simulink subsystem "Plot_Performance"  (R2024b)
settings: Solver=VariableStepAuto  StartTime=0.0  StopTime=10.0  RelTol=1e-3
values from neighbouring files (symbols this model uses):
  BBOD5 = 2    [Run_algo.m]    (also in Run_interpolation.m; perf_plant.m; perf_plant_v3.m; run_bsm1_PIANN.m)
  BNKj_new = 30    [Run_algo.m]    (also in Run_interpolation.m; perf_plant.m; perf_plant_v3.m; run_bsm1_PIANN.m)
  BNO_new = 10    [Run_algo.m]    (also in Run_interpolation.m; perf_plant.m; perf_plant_v3.m; run_bsm1_PIANN.m)
  BSS = 2    [Run_algo.m]    (also in Run_interpolation.m; perf_plant.m; perf_plant_v3.m; run_bsm1_PIANN.m)
  SampleTime = 0.0001    [Run_algo.m]    (also in Run_interpolation.m)
undefined symbols (not defined in the file or in its folder): f_P, i_XB, i_XP
settings Model: Creator=1630327  LastModifiedBy=1630327

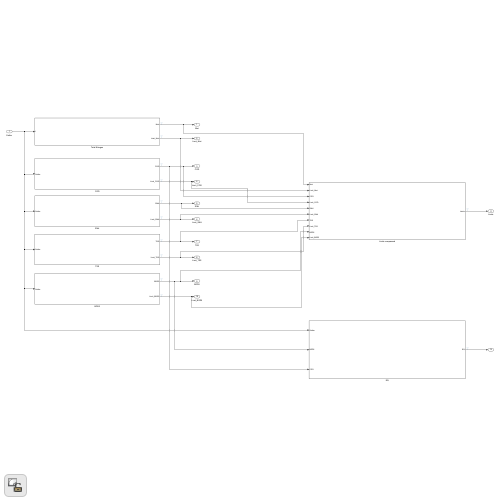
[thumbnail: Simulink's stored preview of the top-level diagram]
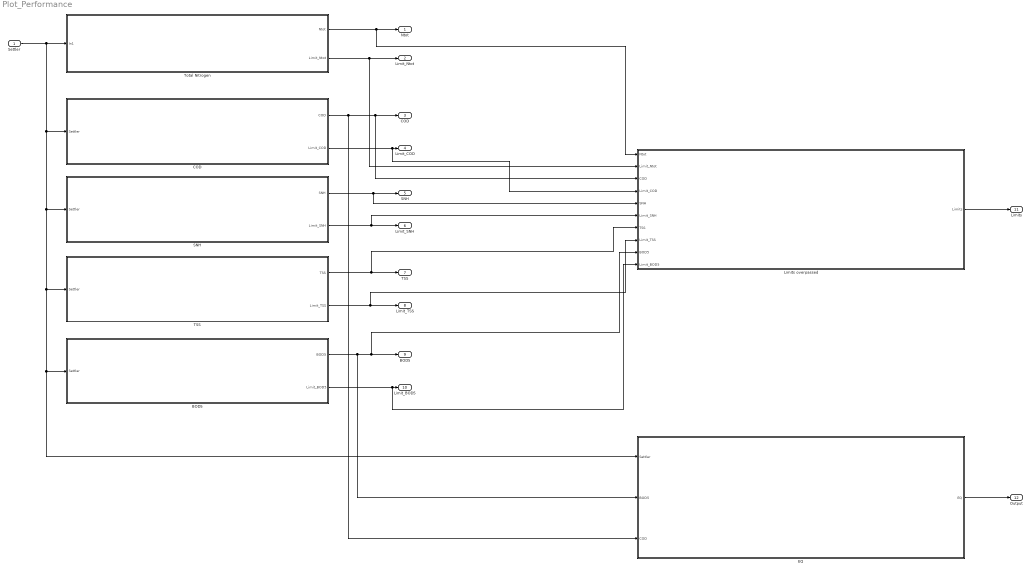
== system Plot_Performance ==
  Settler : Inport
  "BOD5 " : Subsystem
  COD : Subsystem
  EQ : Subsystem
  Limits overpassed : Subsystem
  "SNH " : Subsystem
  "TSS " : Subsystem
  Total Nitrogen : Subsystem
  Ntot : Outport
  Limit_Ntot : Outport  Port=2
  "COD " : Outport  Port=3
  Limit_COD : Outport  Port=4
  SNH : Outport  Port=5
  Limit_SNH : Outport  Port=6
  TSS : Outport  Port=7
  Limit_TSS : Outport  Port=8
  BOD5 : Outport  Port=9
  Limit_BOD5 : Outport  Port=10
  Limits : Outport  Port=11
  Output : Outport  Port=12
  wires:
  Settler/1 -> Total Nitrogen/1(In1), COD/1(Settler), "SNH "/1(Settler), "TSS "/1(Settler), "BOD5 "/1(Settler), EQ/1(Settler)
  Total Nitrogen/1(Ntot) -> Ntot/1, Limits overpassed/1(Ntot)
  Total Nitrogen/2(Limit_Ntot) -> Limit_Ntot/1, Limits overpassed/2(Limit_Ntot)
  COD/1(COD) -> "COD "/1, Limits overpassed/3(COD), EQ/3(COD)
  COD/2(Limit_COD) -> Limit_COD/1, Limits overpassed/4(Limit_COD)
  "SNH "/2(Limit_SNH) -> Limit_SNH/1, Limits overpassed/6(Limit_SNH)
  "SNH "/1(SNH) -> SNH/1, Limits overpassed/5(SNH)
  "TSS "/2(Limit_TSS) -> Limit_TSS/1, Limits overpassed/8(Limit_TSS)
  "TSS "/1(TSS) -> TSS/1, Limits overpassed/7(TSS)
  "BOD5 "/1(BOD5) -> BOD5/1, Limits overpassed/9(BOD5), EQ/2(BOD5)
  "BOD5 "/2(Limit_BOD5) -> Limit_BOD5/1, Limits overpassed/10(Limit_BOD5)
  Limits overpassed/1(Limits) -> Limits/1
  EQ/1(EQ) -> Output/1

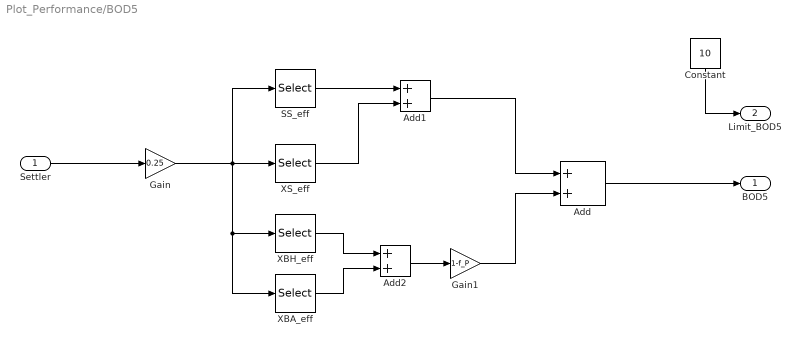
== system Plot_Performance/BOD5  ==
  Settler : Inport
  Add : Sum
  Add1 : Sum
  Add2 : Sum
  Constant : Constant  Value=10  SampleTime=SampleTime
  Gain : Gain  Gain=0.25
  Gain1 : Gain  Gain=1-f_P
  SS_eff : Selector  InputPortWidth=113  IndexOptions=Index vector (dialog)  Indices=[18]  OutputSizes=1
  XBA_eff : Selector  InputPortWidth=113  IndexOptions=Index vector (dialog)  Indices=[22]  OutputSizes=1
  XBH_eff : Selector  InputPortWidth=113  IndexOptions=Index vector (dialog)  Indices=[21]  OutputSizes=1
  XS_eff : Selector  InputPortWidth=113  IndexOptions=Index vector (dialog)  Indices=[20]  OutputSizes=1
  BOD5 : Outport
  Limit_BOD5 : Outport  Port=2
  wires:
  Add1/1 -> Add/1
  Gain1/1 -> Add/2
  Add2/1 -> Gain1/1
  XBA_eff/1 -> Add2/2
  XBH_eff/1 -> Add2/1
  XS_eff/1 -> Add1/2
  SS_eff/1 -> Add1/1
  Gain/1 -> SS_eff/1, XS_eff/1, XBH_eff/1, XBA_eff/1
  Constant/1 -> Limit_BOD5/1
  Add/1 -> BOD5/1
  Settler/1 -> Gain/1

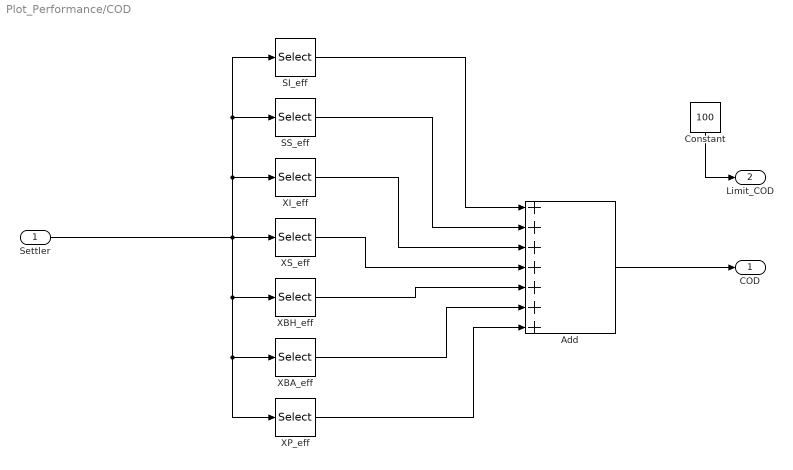
== system Plot_Performance/COD ==
  Settler : Inport
  Add : Sum  Inputs=+++++++
  Constant : Constant  Value=100  SampleTime=SampleTime
  SI_eff : Selector  InputPortWidth=113  IndexOptions=Index vector (dialog)  Indices=[17]  OutputSizes=1
  SS_eff : Selector  InputPortWidth=113  IndexOptions=Index vector (dialog)  Indices=[18]  OutputSizes=1
  XBA_eff : Selector  InputPortWidth=113  IndexOptions=Index vector (dialog)  Indices=[22]  OutputSizes=1
  XBH_eff : Selector  InputPortWidth=113  IndexOptions=Index vector (dialog)  Indices=[21]  OutputSizes=1
  XI_eff : Selector  InputPortWidth=113  IndexOptions=Index vector (dialog)  Indices=[19]  OutputSizes=1
  XP_eff : Selector  InputPortWidth=113  IndexOptions=Index vector (dialog)  Indices=[23]  OutputSizes=1
  XS_eff : Selector  InputPortWidth=113  IndexOptions=Index vector (dialog)  Indices=[20]  OutputSizes=1
  COD : Outport
  Limit_COD : Outport  Port=2
  wires:
  Constant/1 -> Limit_COD/1
  Add/1 -> COD/1
  XP_eff/1 -> Add/7
  XBA_eff/1 -> Add/6
  XBH_eff/1 -> Add/5
  XS_eff/1 -> Add/4
  XI_eff/1 -> Add/3
  SS_eff/1 -> Add/2
  SI_eff/1 -> Add/1
  Settler/1 -> SI_eff/1, SS_eff/1, XI_eff/1, XS_eff/1, XBH_eff/1, XBA_eff/1, XP_eff/1

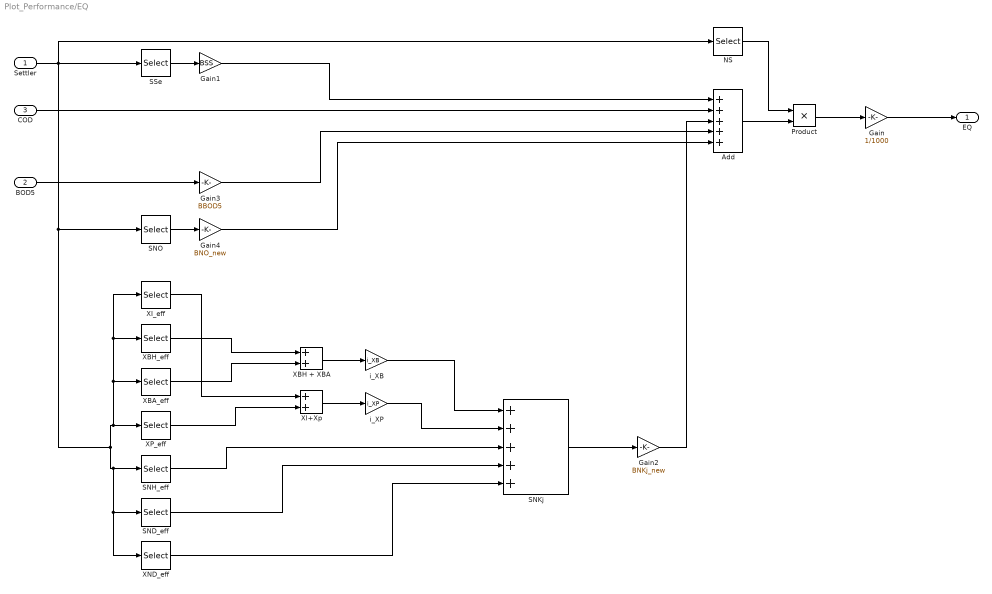
== system Plot_Performance/EQ ==
  Settler : Inport
  BOD5 : Inport  Port=2
  COD : Inport  Port=3
  Add : Sum  Inputs=+++++
  Gain : Gain  Gain=1/1000
  Gain1 : Gain  Gain=BSS
  Gain2 : Gain  Gain=BNKj_new
  Gain3 : Gain  Gain=BBOD5
  Gain4 : Gain  Gain=BNO_new
  NS : Selector  InputPortWidth=113  IndexOptions=Index vector (dialog)  Indices=[31]  OutputSizes=1
  Product : Product
  SND_eff : Selector  InputPortWidth=113  IndexOptions=Index vector (dialog)  Indices=[27]  OutputSizes=1
  SNH_eff : Selector  InputPortWidth=113  IndexOptions=Index vector (dialog)  Indices=[26]  OutputSizes=1
  SNKj : Sum  Inputs=+++++
  SNO : Selector  InputPortWidth=113  IndexOptions=Index vector (dialog)  Indices=[25]  OutputSizes=1
  SSe : Selector  InputPortWidth=113  IndexOptions=Index vector (dialog)  Indices=[30]  OutputSizes=1
  XBA_eff : Selector  InputPortWidth=113  IndexOptions=Index vector (dialog)  Indices=[22]  OutputSizes=1
  XBH + XBA : Sum
  XBH_eff : Selector  InputPortWidth=113  IndexOptions=Index vector (dialog)  Indices=[21]  OutputSizes=1
  XI+Xp : Sum
  XI_eff : Selector  InputPortWidth=113  IndexOptions=Index vector (dialog)  Indices=[19]  OutputSizes=1
  XND_eff : Selector  InputPortWidth=113  IndexOptions=Index vector (dialog)  Indices=[28]  OutputSizes=1
  XP_eff : Selector  InputPortWidth=113  IndexOptions=Index vector (dialog)  Indices=[23]  OutputSizes=1
  i_XB : Gain  Gain=i_XB
  i_XP : Gain  Gain=i_XP
  EQ : Outport
  wires:
  Gain/1 -> EQ/1
  NS/1 -> Product/1
  Product/1 -> Gain/1
  XND_eff/1 -> SNKj/5
  SND_eff/1 -> SNKj/4
  SNH_eff/1 -> SNKj/3
  SNKj/1 -> Gain2/1
  XP_eff/1 -> XI+Xp/2
  i_XP/1 -> SNKj/2
  XI_eff/1 -> XI+Xp/1
  XBH + XBA/1 -> i_XB/1
  XI+Xp/1 -> i_XP/1
  XBH_eff/1 -> XBH + XBA/1
  i_XB/1 -> SNKj/1
  XBA_eff/1 -> XBH + XBA/2
  Add/1 -> Product/2
  Gain4/1 -> Add/5
  SNO/1 -> Gain4/1
  Gain3/1 -> Add/4
  BOD5/1 -> Gain3/1
  Gain2/1 -> Add/3
  Gain1/1 -> Add/1
  COD/1 -> Add/2
  SSe/1 -> Gain1/1
  Settler/1 -> XI_eff/1, XBH_eff/1, XBA_eff/1, XP_eff/1, SNH_eff/1, SND_eff/1, XND_eff/1, SNO/1, SSe/1, NS/1

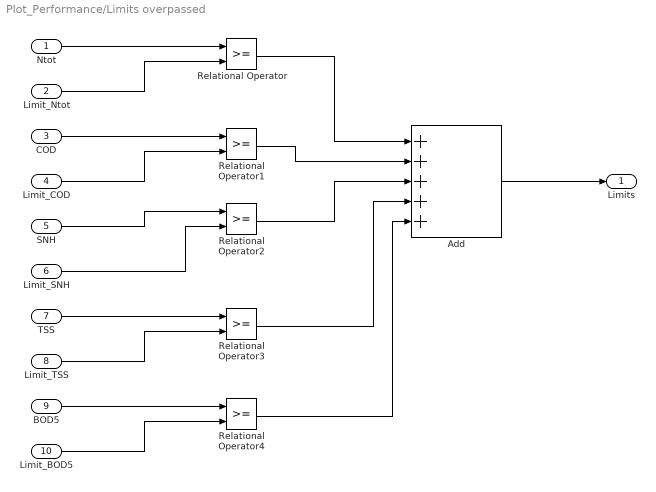
== system Plot_Performance/Limits overpassed ==
  Ntot : Inport
  Limit_Ntot : Inport  Port=2
  COD : Inport  Port=3
  Limit_COD : Inport  Port=4
  SNH : Inport  Port=5
  Limit_SNH : Inport  Port=6
  TSS : Inport  Port=7
  Limit_TSS : Inport  Port=8
  BOD5 : Inport  Port=9
  Limit_BOD5 : Inport  Port=10
  Add : Sum  Inputs=+++++
  Relational Operator{,1..4} (5 alike) : RelationalOperator  OutDataTypeStr=boolean  RndMeth=Simplest  InputSameDT=off
  Limits : Outport
  wires:
  Add/1 -> Limits/1
  Relational Operator4/1 -> Add/5
  Relational Operator3/1 -> Add/4
  Relational Operator2/1 -> Add/3
  Relational Operator1/1 -> Add/2
  Relational Operator/1 -> Add/1
  Limit_BOD5/1 -> Relational Operator4/2
  BOD5/1 -> Relational Operator4/1
  Limit_TSS/1 -> Relational Operator3/2
  TSS/1 -> Relational Operator3/1
  Limit_SNH/1 -> Relational Operator2/2
  SNH/1 -> Relational Operator2/1
  Limit_COD/1 -> Relational Operator1/2
  COD/1 -> Relational Operator1/1
  Limit_Ntot/1 -> Relational Operator/2
  Ntot/1 -> Relational Operator/1

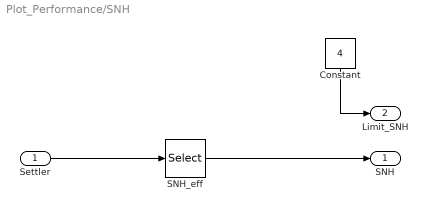
== system Plot_Performance/SNH  ==
  Settler : Inport
  Constant : Constant  Value=4  SampleTime=SampleTime
  SNH_eff : Selector  InputPortWidth=113  IndexOptions=Index vector (dialog)  Indices=[26]  OutputSizes=1
  SNH : Outport
  Limit_SNH : Outport  Port=2
  wires:
  SNH_eff/1 -> SNH/1
  Constant/1 -> Limit_SNH/1
  Settler/1 -> SNH_eff/1

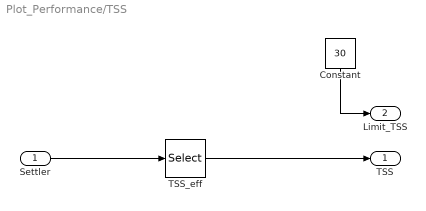
== system Plot_Performance/TSS  ==
  Settler : Inport
  Constant : Constant  Value=30  SampleTime=SampleTime
  TSS_eff : Selector  InputPortWidth=113  IndexOptions=Index vector (dialog)  Indices=[30]  OutputSizes=1
  TSS : Outport
  Limit_TSS : Outport  Port=2
  wires:
  Settler/1 -> TSS_eff/1
  TSS_eff/1 -> TSS/1
  Constant/1 -> Limit_TSS/1

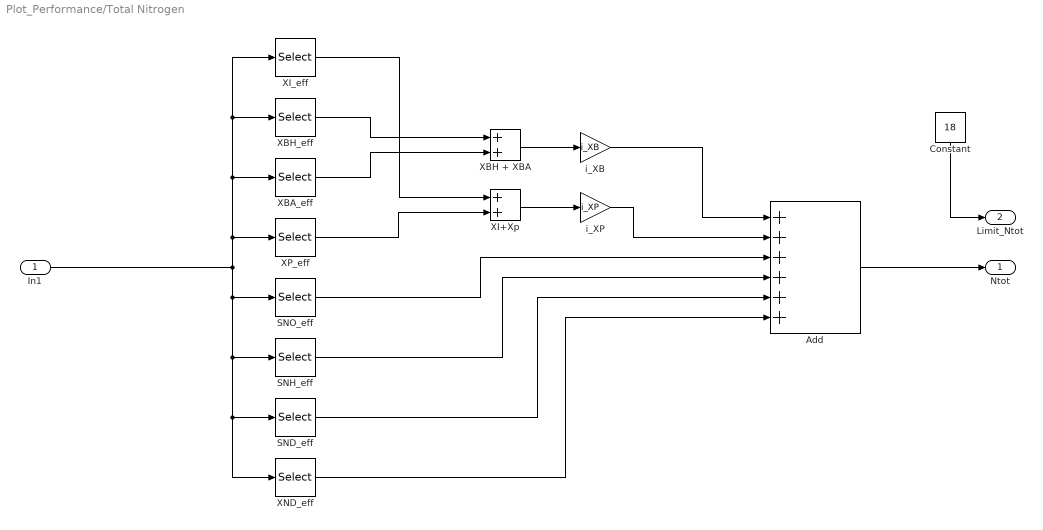
== system Plot_Performance/Total Nitrogen ==
  In1 : Inport
  Add : Sum  Inputs=++++++
  Constant : Constant  Value=18  SampleTime=SampleTime
  SND_eff : Selector  InputPortWidth=113  IndexOptions=Index vector (dialog)  Indices=[27]  OutputSizes=1
  SNH_eff : Selector  InputPortWidth=113  IndexOptions=Index vector (dialog)  Indices=[26]  OutputSizes=1
  SNO_eff : Selector  InputPortWidth=113  IndexOptions=Index vector (dialog)  Indices=[25]  OutputSizes=1
  XBA_eff : Selector  InputPortWidth=113  IndexOptions=Index vector (dialog)  Indices=[22]  OutputSizes=1
  XBH + XBA : Sum
  XBH_eff : Selector  InputPortWidth=113  IndexOptions=Index vector (dialog)  Indices=[21]  OutputSizes=1
  XI+Xp : Sum
  XI_eff : Selector  InputPortWidth=113  IndexOptions=Index vector (dialog)  Indices=[19]  OutputSizes=1
  XND_eff : Selector  InputPortWidth=113  IndexOptions=Index vector (dialog)  Indices=[28]  OutputSizes=1
  XP_eff : Selector  InputPortWidth=113  IndexOptions=Index vector (dialog)  Indices=[23]  OutputSizes=1
  i_XB : Gain  Gain=i_XB
  i_XP : Gain  Gain=i_XP
  Ntot : Outport
  Limit_Ntot : Outport  Port=2
  wires:
  Constant/1 -> Limit_Ntot/1
  Add/1 -> Ntot/1
  XBH_eff/1 -> XBH + XBA/1
  XBA_eff/1 -> XBH + XBA/2
  XI+Xp/1 -> i_XP/1
  i_XP/1 -> Add/2
  XBH + XBA/1 -> i_XB/1
  SNH_eff/1 -> Add/4
  In1/1 -> XI_eff/1, XBH_eff/1, XBA_eff/1, XP_eff/1, SNO_eff/1, SNH_eff/1, SND_eff/1, XND_eff/1
  SNO_eff/1 -> Add/3
  XND_eff/1 -> Add/6
  XI_eff/1 -> XI+Xp/1
  i_XB/1 -> Add/1
  XP_eff/1 -> XI+Xp/2
  SND_eff/1 -> Add/5
